simulink model "asm_dfoc"  (R2021a)
settings: Solver=ode23t  StartTime=0.0  StopTime=1  FixedStep=10^(-4)  MaxStep=1e-8  RelTol=1e-3  EnableMultiTasking=on
InitFcn:
  | clear all;
  | P=4;
  | 
  | Rs=28.5e-3;
  | Rr=15.6e-3;
  | 
  | Lm=8e-3;
  | Lls=306e-6;
  | Llr=232e-6;
  | 
  | J=0.805;
  | B=0;%3.5e-2;
  | Ls = Lls+Lm;
  | Lr = Llr+Lm;
  | 
  | Rt = 0.34;
  | u =6.2922;
  | verim=.97
libraries: pid_lib x5, spsdq0toAlphaBetaZeroLib x1
settings Model: Creator=akcan  LastModifiedBy=MSI-
settings SolverCC: AlgebraicLoopSolver=TrustRegion
settings DataIOCC: LimitDataPoints=on  SaveFormat=Array  SignalLoggingSaveFormat=ModelDataLogs  ReturnWorkspaceOutputs=off
settings OptimizationCC: LifeSpan=inf
settings DebuggingCC: UnderspecifiedInitializationDetection=Classic  MergeDetectMultiDrivingBlocksExec=none  SolverPrmCheckMsg=warning  MultiTaskDSMMsg=warning  MultiTaskCondExecSysMsg=none  SFUnexpectedBacktrackingDiag=warning  SFNoUnconditionalDefaultTransitionDiag=warning  SFExecutionAtInitializationDiag=none  SFMachineParentedDataDiag=warning  ArithmeticOperatorsInVariantConditions=warning
settings HardwareCC: ProdBitPerPointer=32  ProdBitPerSizeT=32  ProdBitPerPtrDiffT=32  ProdLargestAtomicFloat=None  ProdIntDivRoundTo=Undefined  ProdEndianess=Unspecified  ProdWordSize=32  ProdHWDeviceType=32-bit Generic
settings ModelReferenceCC: PropagateSignalLabelsOutOfModel=off
settings SFSimCC: SimUseLocalCustomCode=off  CustomCodeUndefinedFunction=UseInterfaceOnly
settings RTWCC: RTWUseLocalCustomCode=off
settings CodeAppCC: StateflowObjectComments=on
settings GRTTargetCC: TargetLangStandard=C89/C90 (ANSI)
settings ConfigComp: CovMetricSettings=dw  CovSaveCumulativeToWorkspaceVar=on  CovSaveSingleToWorkspaceVar=on  CovExternalEMLEnable=off
settings SimscapeCC: SimscapeNormalizeSystem=off

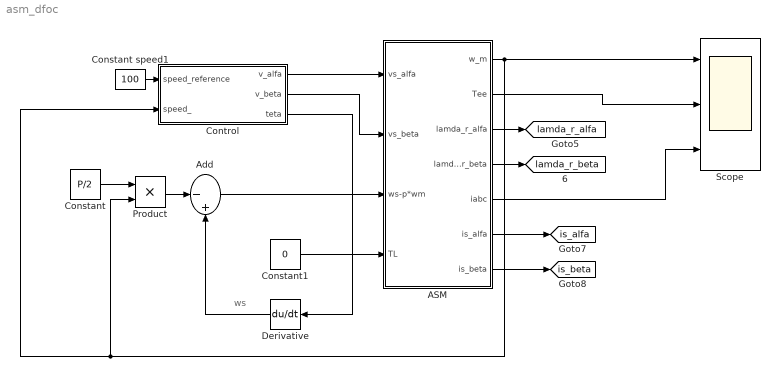
== system asm_dfoc ==
  note: ws
  ASM : Subsystem
  Add : Sum  Inputs=|-+
  Constant : Constant  Value=P/2
  Constant speed1 : Constant  Value=100
  Constant1 : Constant  Value=0
  Control : Subsystem
  Derivative : Derivative
  Product : Product
  Scope : Scope  NumInputPorts=3
  tag scope: is_alfa=global, is_beta=global, lamda_r_alfa=global, lamda_r_beta=global
  wires:
  ASM/3(lamda_r_alfa) -> [lamda_r_alfa]
  ASM/4(lamda_r_beta) -> [lamda_r_beta]
  Control/1("v_alfa ") -> ASM/1(vs_alfa)
  Product/1 -> Add/1
  Constant/1 -> Product/1
  ASM/1(w_m) -> Control/2(speed_), Product/2, Scope/1
  Derivative/1 -> Add/2
  Constant1/1 -> ASM/4(TL)
  Control/2(v_beta) -> ASM/2(vs_beta)
  ASM/7(is_beta) -> [is_beta]
  ASM/6(is_alfa) -> [is_alfa]
  Add/1 -> ASM/3("ws-p*wm ")
  Control/3(teta) -> Derivative/1
  Constant speed1/1 -> Control/1(speed_reference)
  ASM/2(Tee) -> Scope/2
  ASM/5(iabc) -> Scope/3

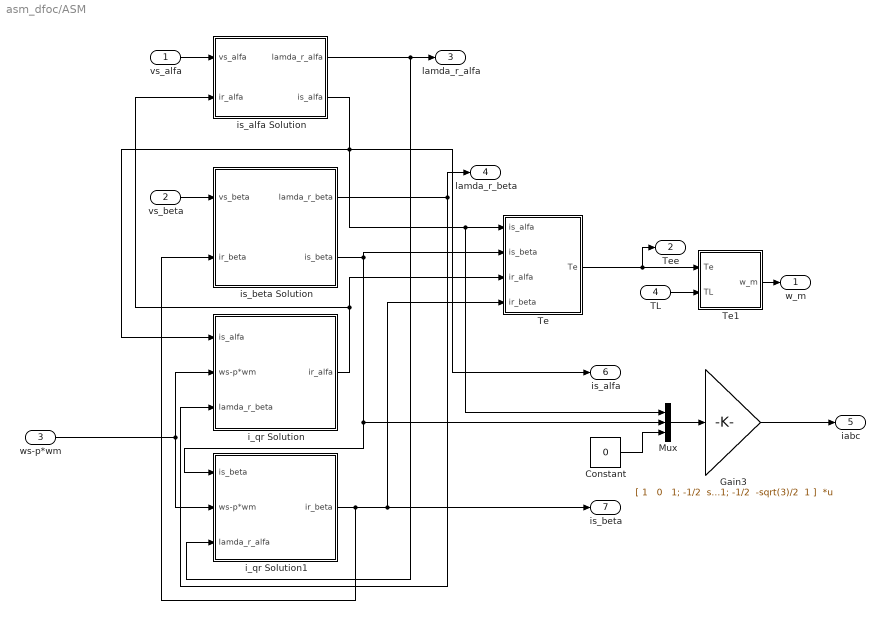
== system asm_dfoc/ASM ==
  vs_alfa : Inport
  vs_beta : Inport  Port=2
  "ws-p*wm " : Inport  Port=3
  TL : Inport  Port=4
  Constant : Constant  Value=0
  Gain3 : Gain  Gain="[ 1   0   1; -1/2  sqrt(3)/2   1; -1/2  -sqrt(3)/2  1 ]"  Multiplication=Matrix(K*u) (u vector)  SaturateOnIntegerOverflow=on  OutDataTypeStr=Inherit: Same as input  ParamDataTypeStr=Inherit: Same as input
  Mux : Mux  Inputs=3
  Te : Subsystem
  Te1 : Subsystem
  i_qr Solution : Subsystem
  i_qr Solution1 : Subsystem
  is_alfa Solution : Subsystem
  is_beta Solution : Subsystem
  w_m : Outport
  Tee : Outport  Port=2
  lamda_r_alfa : Outport  Port=3
  lamda_r_beta : Outport  Port=4
  iabc : Outport  Port=5
  is_alfa : Outport  Port=6
  is_beta : Outport  Port=7
  wires:
  vs_alfa/1 -> is_alfa Solution/1(vs_alfa)
  TL/1 -> Te1/2(TL)
  Te1/1(w_m) -> w_m/1
  Te/1(Te) -> Tee/1, Te1/1(Te)
  vs_beta/1 -> is_beta Solution/1(vs_beta)
  "ws-p*wm "/1 -> i_qr Solution1/2(ws-p*wm), i_qr Solution/2(ws-p*wm)
  Gain3/1 -> iabc/1
  Mux/1 -> Gain3/1
  Constant/1 -> Mux/3
  is_alfa Solution/1(lamda_r_alfa) -> i_qr Solution1/3(lamda_r_alfa), lamda_r_alfa/1
  is_beta Solution/1(lamda_r_beta) -> lamda_r_beta/1, i_qr Solution/3(lamda_r_beta)
  i_qr Solution/1(ir_alfa) -> Te/3(ir_alfa), is_alfa Solution/2(ir_alfa)
  is_beta Solution/2(is_beta) -> Mux/2, i_qr Solution1/1(is_beta), Te/2(is_beta)
  i_qr Solution1/1(ir_beta) -> is_beta/1, Te/4(ir_beta), is_beta Solution/2(ir_beta)
  is_alfa Solution/2(is_alfa) -> is_alfa/1, Mux/1, Te/1(is_alfa), i_qr Solution/1(is_alfa)

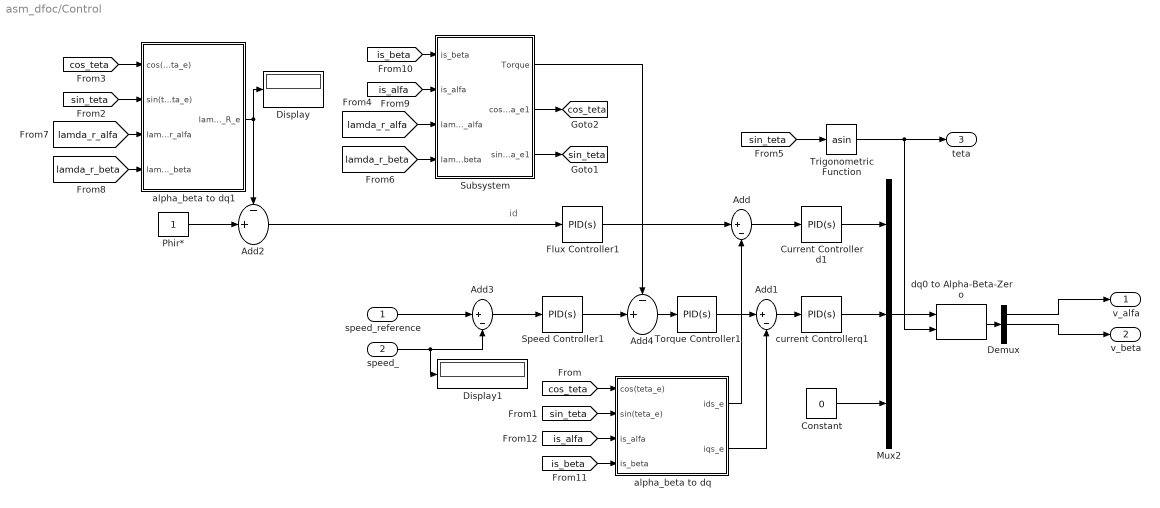
== system asm_dfoc/Control ==
  note: id
  speed_reference : Inport
  speed_ : Inport  Port=2
  Add : Sum  Inputs=|+-
  Add1 : Sum  Inputs=|+-
  Add2 : Sum  Inputs=-+|
  Add3 : Sum  Inputs=|+-
  Add4 : Sum  Inputs=-+|
  Constant : Constant  Value=0
  Current Controller d1 : pid_lib/PID Controller  Controller=PID  Form=Parallel  TimeDomain=Continuous-time  UseExternalTs=off  SampleTime=1  IntegratorMethod=Forward Euler  FilterMethod=Forward Euler  ControllerParametersSource=internal  P=1  I=0.001  D=0  UseFilter=on  N=100  TunerSelectOption=Transfer Function Based (PID Tuner App)  InitialConditionSource=internal  InitialConditionForIntegrator=50  InitialConditionForFilter=0  DifferentiatorICPrevScaledInput=0  ExternalReset=none  TrackingMode=off  Kt=1  LimitOutput=on  SatLimitsSource=internal  UpperSaturationLimit=600  LowerSaturationLimit=-600  LinearizeAsGain=off  AntiWindupMode=clamping  Kb=1  POutMin=[]  POutMax=[]  IOutMin=[]  IOutMax=[]  DOutMin=[]  DOutMax=[]  NOutMin=[]  NOutMax=[]  SumOutMin=[]  SumOutMax=[]  SaturationOutMin=[]  SaturationOutMax=[]  PParamMin=[]  PParamMax=[]  IParamMin=[]  IParamMax=[]  DParamMin=[]  DParamMax=[]  NParamMin=[]  NParamMax=[]  KbParamMin=[]  KbParamMax=[]  KtParamMin=[]  KtParamMax=[]  KbOutMin=[]  KbOutMax=[]  KtOutMin=[]  KtOutMax=[]  IntegratorOutMin=[]  IntegratorOutMax=[]  FilterOutMin=[]  FilterOutMax=[]  SumI1OutMin=[]  SumI1OutMax=[]  SumI2OutMin=[]  SumI2OutMax=[]  SumI3OutMin=[]  SumI3OutMax=[]  SumI4OutMin=[]  SumI4OutMax=[]  SumDOutMin=[]  SumDOutMax=[]  DifferentiatorOutMin=[]  DifferentiatorOutMax=[]  FilterDiffOutCoefMin=[]  FilterDiffOutCoefMax=[]  ReciprocalOutMin=[]  ReciprocalOutMax=[]  SumDenOutMin=[]  SumDenOutMax=[]  SumNumOutMin=[]  SumNumOutMax=[]  DivideOutMin=[]  DivideOutMax=[]  UdiffTsProdOutMin=[]  UdiffTsProdOutMax=[]  NTsProdOutMin=[]  NTsProdOutMax=[]  UintegralTsProdOutMin=[]  UintegralTsProdOutMax=[]  UngainTsProdOutMin=[]  UngainTsProdOutMax=[]  IntegratorContinuousStateAttributes=''  IntegratorStateMustResolveToSignalObject=off  IntegratorRTWStateStorageClass=Auto  FilterContinuousStateAttributes=''  FilterStateMustResolveToSignalObject=off  FilterRTWStateStorageClass=Auto  ParallelPVariant=InternalParameters  IdealPVariant=Disabled  IVariant=InternalParameters  DVariant=InternalParameters  IntegratorVariant=Continuous  SatVariant=Enabled  AWVariant=ContClampingParallel  PCopyVariant=Disabled  TRVariant=Disabled  FdbkBlocksVariant=Forward  IdealPFdbkVariant=Disabled  SatFdbkVariant=Disabled  DerivativeFilterVariant=ContFilter  NVariant=InternalParameters  NCopyVariant=Disabled  FilterICVariant=InternalICsFilter  IntegratorICVariant=InternalICs  ExternalResetVariant=Disabled  TRSumVariant=Passthrough  SumFdbkVariant=Disabled  SumVariant=Sum_PID  TsampFilterVariant=InternalTs  TsampNgainVariant=Passthrough  TsampIntegralVariant=Passthrough  ExternalSaturationOutDataTypeStr=Inherit: Same as second input
  Demux : Demux  Outputs=3
  Display : Display
  Display1 : Display
  Flux Controller1 : pid_lib/PID Controller  Controller=PID  Form=Parallel  TimeDomain=Continuous-time  UseExternalTs=off  SampleTime=1  IntegratorMethod=Forward Euler  FilterMethod=Forward Euler  ControllerParametersSource=internal  P=1  I=0.001  D=0  UseFilter=on  N=100  TunerSelectOption=Transfer Function Based (PID Tuner App)  InitialConditionSource=internal  InitialConditionForIntegrator=100  InitialConditionForFilter=0  DifferentiatorICPrevScaledInput=0  ExternalReset=none  TrackingMode=off  Kt=1  LimitOutput=on  SatLimitsSource=internal  UpperSaturationLimit=300  LowerSaturationLimit=-300  LinearizeAsGain=off  AntiWindupMode=clamping  Kb=1  POutMin=[]  POutMax=[]  IOutMin=[]  IOutMax=[]  DOutMin=[]  DOutMax=[]  NOutMin=[]  NOutMax=[]  SumOutMin=[]  SumOutMax=[]  SaturationOutMin=[]  SaturationOutMax=[]  PParamMin=[]  PParamMax=[]  IParamMin=[]  IParamMax=[]  DParamMin=[]  DParamMax=[]  NParamMin=[]  NParamMax=[]  KbParamMin=[]  KbParamMax=[]  KtParamMin=[]  KtParamMax=[]  KbOutMin=[]  KbOutMax=[]  KtOutMin=[]  KtOutMax=[]  IntegratorOutMin=[]  IntegratorOutMax=[]  FilterOutMin=[]  FilterOutMax=[]  SumI1OutMin=[]  SumI1OutMax=[]  SumI2OutMin=[]  SumI2OutMax=[]  SumI3OutMin=[]  SumI3OutMax=[]  SumI4OutMin=[]  SumI4OutMax=[]  SumDOutMin=[]  SumDOutMax=[]  DifferentiatorOutMin=[]  DifferentiatorOutMax=[]  FilterDiffOutCoefMin=[]  FilterDiffOutCoefMax=[]  ReciprocalOutMin=[]  ReciprocalOutMax=[]  SumDenOutMin=[]  SumDenOutMax=[]  SumNumOutMin=[]  SumNumOutMax=[]  DivideOutMin=[]  DivideOutMax=[]  UdiffTsProdOutMin=[]  UdiffTsProdOutMax=[]  NTsProdOutMin=[]  NTsProdOutMax=[]  UintegralTsProdOutMin=[]  UintegralTsProdOutMax=[]  UngainTsProdOutMin=[]  UngainTsProdOutMax=[]  IntegratorContinuousStateAttributes=''  IntegratorStateMustResolveToSignalObject=off  IntegratorRTWStateStorageClass=Auto  FilterContinuousStateAttributes=''  FilterStateMustResolveToSignalObject=off  FilterRTWStateStorageClass=Auto  ParallelPVariant=InternalParameters  IdealPVariant=Disabled  IVariant=InternalParameters  DVariant=InternalParameters  IntegratorVariant=Continuous  SatVariant=Enabled  AWVariant=ContClampingParallel  PCopyVariant=Disabled  TRVariant=Disabled  FdbkBlocksVariant=Forward  IdealPFdbkVariant=Disabled  SatFdbkVariant=Disabled  DerivativeFilterVariant=ContFilter  NVariant=InternalParameters  NCopyVariant=Disabled  FilterICVariant=InternalICsFilter  IntegratorICVariant=InternalICs  ExternalResetVariant=Disabled  TRSumVariant=Passthrough  SumFdbkVariant=Disabled  SumVariant=Sum_PID  TsampFilterVariant=InternalTs  TsampNgainVariant=Passthrough  TsampIntegralVariant=Passthrough  ExternalSaturationOutDataTypeStr=Inherit: Same as second input
  Mux2 : Mux  Inputs=3
  Phir* : Constant
  Speed Controller1 : pid_lib/PID Controller  Controller=PID  Form=Parallel  TimeDomain=Continuous-time  UseExternalTs=off  SampleTime=1  IntegratorMethod=Forward Euler  FilterMethod=Forward Euler  ControllerParametersSource=internal  P=1  I=0.01  D=0  UseFilter=on  N=100  TunerSelectOption=Transfer Function Based (PID Tuner App)  InitialConditionSource=internal  InitialConditionForIntegrator=100  InitialConditionForFilter=0  DifferentiatorICPrevScaledInput=0  ExternalReset=none  TrackingMode=off  Kt=1  LimitOutput=off  SatLimitsSource=internal  UpperSaturationLimit=200  LowerSaturationLimit=-200  LinearizeAsGain=off  AntiWindupMode=clamping  Kb=1  POutMin=[]  POutMax=[]  IOutMin=[]  IOutMax=[]  DOutMin=[]  DOutMax=[]  NOutMin=[]  NOutMax=[]  SumOutMin=[]  SumOutMax=[]  SaturationOutMin=[]  SaturationOutMax=[]  PParamMin=[]  PParamMax=[]  IParamMin=[]  IParamMax=[]  DParamMin=[]  DParamMax=[]  NParamMin=[]  NParamMax=[]  KbParamMin=[]  KbParamMax=[]  KtParamMin=[]  KtParamMax=[]  KbOutMin=[]  KbOutMax=[]  KtOutMin=[]  KtOutMax=[]  IntegratorOutMin=[]  IntegratorOutMax=[]  FilterOutMin=[]  FilterOutMax=[]  SumI1OutMin=[]  SumI1OutMax=[]  SumI2OutMin=[]  SumI2OutMax=[]  SumI3OutMin=[]  SumI3OutMax=[]  SumI4OutMin=[]  SumI4OutMax=[]  SumDOutMin=[]  SumDOutMax=[]  DifferentiatorOutMin=[]  DifferentiatorOutMax=[]  FilterDiffOutCoefMin=[]  FilterDiffOutCoefMax=[]  ReciprocalOutMin=[]  ReciprocalOutMax=[]  SumDenOutMin=[]  SumDenOutMax=[]  SumNumOutMin=[]  SumNumOutMax=[]  DivideOutMin=[]  DivideOutMax=[]  UdiffTsProdOutMin=[]  UdiffTsProdOutMax=[]  NTsProdOutMin=[]  NTsProdOutMax=[]  UintegralTsProdOutMin=[]  UintegralTsProdOutMax=[]  UngainTsProdOutMin=[]  UngainTsProdOutMax=[]  IntegratorContinuousStateAttributes=''  IntegratorStateMustResolveToSignalObject=off  IntegratorRTWStateStorageClass=Auto  FilterContinuousStateAttributes=''  FilterStateMustResolveToSignalObject=off  FilterRTWStateStorageClass=Auto  ParallelPVariant=InternalParameters  IdealPVariant=Disabled  IVariant=InternalParameters  DVariant=InternalParameters  IntegratorVariant=Continuous  SatVariant=Disabled  AWVariant=Passthrough  PCopyVariant=Disabled  TRVariant=Disabled  FdbkBlocksVariant=Forward  IdealPFdbkVariant=Disabled  SatFdbkVariant=Disabled  DerivativeFilterVariant=ContFilter  NVariant=InternalParameters  NCopyVariant=Disabled  FilterICVariant=InternalICsFilter  IntegratorICVariant=InternalICs  ExternalResetVariant=Disabled  TRSumVariant=Passthrough  SumFdbkVariant=Disabled  SumVariant=Sum_PID  TsampFilterVariant=InternalTs  TsampNgainVariant=Passthrough  TsampIntegralVariant=Passthrough  ExternalSaturationOutDataTypeStr=Inherit: Same as second input
  Subsystem : Subsystem
  Torque Controller1 : pid_lib/PID Controller  Controller=PID  Form=Parallel  TimeDomain=Continuous-time  UseExternalTs=off  SampleTime=1  IntegratorMethod=Forward Euler  FilterMethod=Forward Euler  ControllerParametersSource=internal  P=1  I=0.01  D=0  UseFilter=on  N=100  TunerSelectOption=Transfer Function Based (PID Tuner App)  InitialConditionSource=internal  InitialConditionForIntegrator=50  InitialConditionForFilter=0  DifferentiatorICPrevScaledInput=0  ExternalReset=none  TrackingMode=off  Kt=1  LimitOutput=on  SatLimitsSource=internal  UpperSaturationLimit=300  LowerSaturationLimit=-300  LinearizeAsGain=off  AntiWindupMode=clamping  Kb=1  POutMin=[]  POutMax=[]  IOutMin=[]  IOutMax=[]  DOutMin=[]  DOutMax=[]  NOutMin=[]  NOutMax=[]  SumOutMin=[]  SumOutMax=[]  SaturationOutMin=[]  SaturationOutMax=[]  PParamMin=[]  PParamMax=[]  IParamMin=[]  IParamMax=[]  DParamMin=[]  DParamMax=[]  NParamMin=[]  NParamMax=[]  KbParamMin=[]  KbParamMax=[]  KtParamMin=[]  KtParamMax=[]  KbOutMin=[]  KbOutMax=[]  KtOutMin=[]  KtOutMax=[]  IntegratorOutMin=[]  IntegratorOutMax=[]  FilterOutMin=[]  FilterOutMax=[]  SumI1OutMin=[]  SumI1OutMax=[]  SumI2OutMin=[]  SumI2OutMax=[]  SumI3OutMin=[]  SumI3OutMax=[]  SumI4OutMin=[]  SumI4OutMax=[]  SumDOutMin=[]  SumDOutMax=[]  DifferentiatorOutMin=[]  DifferentiatorOutMax=[]  FilterDiffOutCoefMin=[]  FilterDiffOutCoefMax=[]  ReciprocalOutMin=[]  ReciprocalOutMax=[]  SumDenOutMin=[]  SumDenOutMax=[]  SumNumOutMin=[]  SumNumOutMax=[]  DivideOutMin=[]  DivideOutMax=[]  UdiffTsProdOutMin=[]  UdiffTsProdOutMax=[]  NTsProdOutMin=[]  NTsProdOutMax=[]  UintegralTsProdOutMin=[]  UintegralTsProdOutMax=[]  UngainTsProdOutMin=[]  UngainTsProdOutMax=[]  IntegratorContinuousStateAttributes=''  IntegratorStateMustResolveToSignalObject=off  IntegratorRTWStateStorageClass=Auto  FilterContinuousStateAttributes=''  FilterStateMustResolveToSignalObject=off  FilterRTWStateStorageClass=Auto  ParallelPVariant=InternalParameters  IdealPVariant=Disabled  IVariant=InternalParameters  DVariant=InternalParameters  IntegratorVariant=Continuous  SatVariant=Enabled  AWVariant=ContClampingParallel  PCopyVariant=Disabled  TRVariant=Disabled  FdbkBlocksVariant=Forward  IdealPFdbkVariant=Disabled  SatFdbkVariant=Disabled  DerivativeFilterVariant=ContFilter  NVariant=InternalParameters  NCopyVariant=Disabled  FilterICVariant=InternalICsFilter  IntegratorICVariant=InternalICs  ExternalResetVariant=Disabled  TRSumVariant=Passthrough  SumFdbkVariant=Disabled  SumVariant=Sum_PID  TsampFilterVariant=InternalTs  TsampNgainVariant=Passthrough  TsampIntegralVariant=Passthrough  ExternalSaturationOutDataTypeStr=Inherit: Same as second input
  Trigonometric Function : Trigonometry  Operator=asin
  alpha_beta to dq : Subsystem
  alpha_beta to dq1 : Subsystem
  current Controllerq1 : pid_lib/PID Controller  Controller=PID  Form=Parallel  TimeDomain=Continuous-time  UseExternalTs=off  SampleTime=1  IntegratorMethod=Forward Euler  FilterMethod=Forward Euler  ControllerParametersSource=internal  P=1  I=0.01  D=0  UseFilter=on  N=100  TunerSelectOption=Transfer Function Based (PID Tuner App)  InitialConditionSource=internal  InitialConditionForIntegrator=50  InitialConditionForFilter=0  DifferentiatorICPrevScaledInput=0  ExternalReset=none  TrackingMode=off  Kt=1  LimitOutput=on  SatLimitsSource=internal  UpperSaturationLimit=600  LowerSaturationLimit=-600  LinearizeAsGain=off  AntiWindupMode=clamping  Kb=1  POutMin=[]  POutMax=[]  IOutMin=[]  IOutMax=[]  DOutMin=[]  DOutMax=[]  NOutMin=[]  NOutMax=[]  SumOutMin=[]  SumOutMax=[]  SaturationOutMin=[]  SaturationOutMax=[]  PParamMin=[]  PParamMax=[]  IParamMin=[]  IParamMax=[]  DParamMin=[]  DParamMax=[]  NParamMin=[]  NParamMax=[]  KbParamMin=[]  KbParamMax=[]  KtParamMin=[]  KtParamMax=[]  KbOutMin=[]  KbOutMax=[]  KtOutMin=[]  KtOutMax=[]  IntegratorOutMin=[]  IntegratorOutMax=[]  FilterOutMin=[]  FilterOutMax=[]  SumI1OutMin=[]  SumI1OutMax=[]  SumI2OutMin=[]  SumI2OutMax=[]  SumI3OutMin=[]  SumI3OutMax=[]  SumI4OutMin=[]  SumI4OutMax=[]  SumDOutMin=[]  SumDOutMax=[]  DifferentiatorOutMin=[]  DifferentiatorOutMax=[]  FilterDiffOutCoefMin=[]  FilterDiffOutCoefMax=[]  ReciprocalOutMin=[]  ReciprocalOutMax=[]  SumDenOutMin=[]  SumDenOutMax=[]  SumNumOutMin=[]  SumNumOutMax=[]  DivideOutMin=[]  DivideOutMax=[]  UdiffTsProdOutMin=[]  UdiffTsProdOutMax=[]  NTsProdOutMin=[]  NTsProdOutMax=[]  UintegralTsProdOutMin=[]  UintegralTsProdOutMax=[]  UngainTsProdOutMin=[]  UngainTsProdOutMax=[]  IntegratorContinuousStateAttributes=''  IntegratorStateMustResolveToSignalObject=off  IntegratorRTWStateStorageClass=Auto  FilterContinuousStateAttributes=''  FilterStateMustResolveToSignalObject=off  FilterRTWStateStorageClass=Auto  ParallelPVariant=InternalParameters  IdealPVariant=Disabled  IVariant=InternalParameters  DVariant=InternalParameters  IntegratorVariant=Continuous  SatVariant=Enabled  AWVariant=ContClampingParallel  PCopyVariant=Disabled  TRVariant=Disabled  FdbkBlocksVariant=Forward  IdealPFdbkVariant=Disabled  SatFdbkVariant=Disabled  DerivativeFilterVariant=ContFilter  NVariant=InternalParameters  NCopyVariant=Disabled  FilterICVariant=InternalICsFilter  IntegratorICVariant=InternalICs  ExternalResetVariant=Disabled  TRSumVariant=Passthrough  SumFdbkVariant=Disabled  SumVariant=Sum_PID  TsampFilterVariant=InternalTs  TsampNgainVariant=Passthrough  TsampIntegralVariant=Passthrough  ExternalSaturationOutDataTypeStr=Inherit: Same as second input
  dq0 to Alpha-Beta-Zero : spsdq0toAlphaBetaZeroLib/dq0 to Alpha-Beta-Zero  Alignment=Aligned with phase A axis
      settings: SourceProductBaseCode=PS
  "v_alfa " : Outport
  v_beta : Outport  Port=2
  teta : Outport  Port=3
  tag scope: cos_teta=global, sin_teta=global
  wires:
  Demux/2 -> v_beta/1
  Phir*/1 -> Add2/2
  Add4/1 -> Torque Controller1/1
  Add2/1 -> Flux Controller1/1
  speed_reference/1 -> Add3/1
  Speed Controller1/1 -> Add4/2
  Add/1 -> Current Controller d1/1
  Add1/1 -> current Controllerq1/1
  Mux2/1 -> dq0 to Alpha-Beta-Zero/1
  Constant/1 -> Mux2/3
  dq0 to Alpha-Beta-Zero/1 -> Demux/1
  Demux/1 -> "v_alfa "/1
  Trigonometric Function/1 -> teta/1, dq0 to Alpha-Beta-Zero/2
  alpha_beta to dq1/1("lamda_R_e ") -> Add2/1, Display/1
  alpha_beta to dq/1("ids_e ") -> Add/2
  alpha_beta to dq/2(iqs_e) -> Add1/2
  Flux Controller1/1 -> Add/1
  Torque Controller1/1 -> Add1/1
  Current Controller d1/1 -> Mux2/1
  current Controllerq1/1 -> Mux2/2
  Subsystem/3(sin_teta_e1) -> [sin_teta]
  Subsystem/2(cos_teta_e1) -> [cos_teta]
  [cos_teta] -> alpha_beta to dq/1(cos(teta_e))
  [sin_teta] -> alpha_beta to dq/2(sin(teta_e))
  [sin_teta] -> alpha_beta to dq1/2(sin(teta_e))
  [cos_teta] -> alpha_beta to dq1/1(cos(teta_e))
  [lamda_r_alfa] -> Subsystem/3("lamda_r_alfa ")
  [sin_teta] -> Trigonometric Function/1
  [lamda_r_beta] -> Subsystem/4(lamda_r_beta)
  [lamda_r_alfa] -> alpha_beta to dq1/3(lamda_r_alfa)
  [lamda_r_beta] -> alpha_beta to dq1/4(lamda_r_beta)
  [is_alfa] -> Subsystem/2(is_alfa)
  [is_beta] -> Subsystem/1(is_beta)
  [is_beta] -> alpha_beta to dq/4(is_beta)
  [is_alfa] -> alpha_beta to dq/3(is_alfa)
  speed_/1 -> Display1/1, Add3/2
  Add3/1 -> Speed Controller1/1
  Subsystem/1(Torque) -> Add4/1

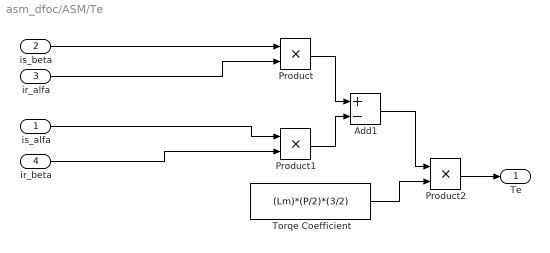
== system asm_dfoc/ASM/Te ==
  is_alfa : Inport
  is_beta : Inport  Port=2
  ir_alfa : Inport  Port=3
  ir_beta : Inport  Port=4
  Add1 : Sum  Inputs=+-
  Product : Product
  Product1 : Product
  Product2 : Product
  Torqe Coefficient : Constant  Value=(Lm)*(P/2)*(3/2)
  Te : Outport
  wires:
  Product/1 -> Add1/1
  Product1/1 -> Add1/2
  Add1/1 -> Product2/1
  Torqe Coefficient/1 -> Product2/2
  Product2/1 -> Te/1
  is_beta/1 -> Product/1
  ir_alfa/1 -> Product/2
  is_alfa/1 -> Product1/1
  ir_beta/1 -> Product1/2

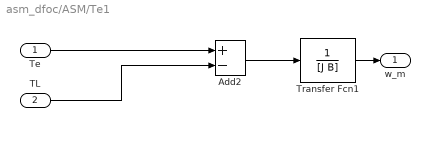
== system asm_dfoc/ASM/Te1 ==
  Te : Inport
  TL : Inport  Port=2
  Add2 : Sum  Inputs=+-
  Transfer Fcn1 : TransferFcn  Denominator=[J B]
  w_m : Outport
  wires:
  Add2/1 -> Transfer Fcn1/1
  Transfer Fcn1/1 -> w_m/1
  Te/1 -> Add2/1
  TL/1 -> Add2/2

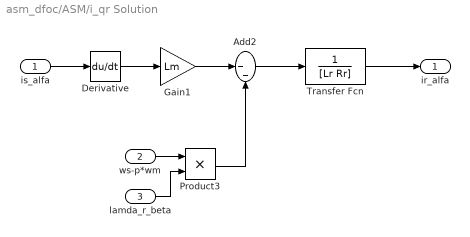
== system asm_dfoc/ASM/i_qr Solution ==
  is_alfa : Inport
  ws-p*wm : Inport  Port=2
  lamda_r_beta : Inport  Port=3
  Add2 : Sum  Inputs=|--
  Derivative : Derivative
  Gain1 : Gain  Gain=Lm
  Product3 : Product
  Transfer Fcn : TransferFcn  Denominator=[Lr Rr]
  ir_alfa : Outport
  wires:
  is_alfa/1 -> Derivative/1
  Derivative/1 -> Gain1/1
  Gain1/1 -> Add2/1
  Product3/1 -> Add2/2
  ws-p*wm/1 -> Product3/1
  lamda_r_beta/1 -> Product3/2
  Add2/1 -> Transfer Fcn/1
  Transfer Fcn/1 -> ir_alfa/1

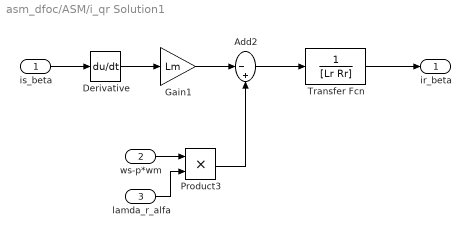
== system asm_dfoc/ASM/i_qr Solution1 ==
  is_beta : Inport
  ws-p*wm : Inport  Port=2
  lamda_r_alfa : Inport  Port=3
  Add2 : Sum  Inputs=|-+
  Derivative : Derivative
  Gain1 : Gain  Gain=Lm
  Product3 : Product
  Transfer Fcn : TransferFcn  Denominator=[Lr Rr]
  ir_beta : Outport
  wires:
  is_beta/1 -> Derivative/1
  Derivative/1 -> Gain1/1
  Gain1/1 -> Add2/1
  Product3/1 -> Add2/2
  ws-p*wm/1 -> Product3/1
  lamda_r_alfa/1 -> Product3/2
  Add2/1 -> Transfer Fcn/1
  Transfer Fcn/1 -> ir_beta/1

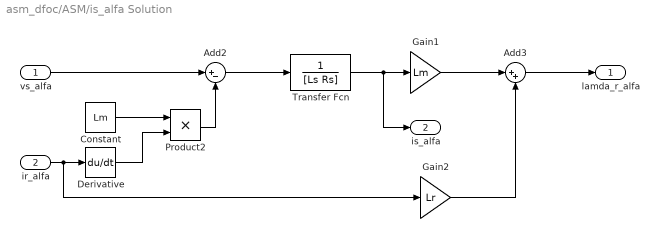
== system asm_dfoc/ASM/is_alfa Solution ==
  vs_alfa : Inport
  ir_alfa : Inport  Port=2
  Add2 : Sum  Inputs=|+-
  Add3 : Sum  Inputs=|++
  Constant : Constant  Value=Lm
  Derivative : Derivative
  Gain1 : Gain  Gain=Lm
  Gain2 : Gain  Gain=Lr
  Product2 : Product
  Transfer Fcn : TransferFcn  Denominator=[Ls Rs]
  lamda_r_alfa : Outport
  is_alfa : Outport  Port=2
  wires:
  vs_alfa/1 -> Add2/1
  Product2/1 -> Add2/2
  Add2/1 -> Transfer Fcn/1
  Transfer Fcn/1 -> Gain1/1, is_alfa/1
  Constant/1 -> Product2/1
  ir_alfa/1 -> Gain2/1, Derivative/1
  Derivative/1 -> Product2/2
  Gain1/1 -> Add3/1
  Gain2/1 -> Add3/2
  Add3/1 -> lamda_r_alfa/1

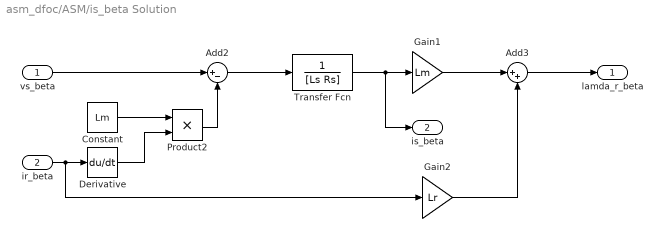
== system asm_dfoc/ASM/is_beta Solution ==
  vs_beta : Inport
  ir_beta : Inport  Port=2
  Add2 : Sum  Inputs=|+-
  Add3 : Sum  Inputs=|++
  Constant : Constant  Value=Lm
  Derivative : Derivative
  Gain1 : Gain  Gain=Lm
  Gain2 : Gain  Gain=Lr
  Product2 : Product
  Transfer Fcn : TransferFcn  Denominator=[Ls Rs]
  lamda_r_beta : Outport
  is_beta : Outport  Port=2
  wires:
  vs_beta/1 -> Add2/1
  Product2/1 -> Add2/2
  Add2/1 -> Transfer Fcn/1
  Transfer Fcn/1 -> Gain1/1, is_beta/1
  Constant/1 -> Product2/1
  ir_beta/1 -> Gain2/1, Derivative/1
  Derivative/1 -> Product2/2
  Gain1/1 -> Add3/1
  Gain2/1 -> Add3/2
  Add3/1 -> lamda_r_beta/1

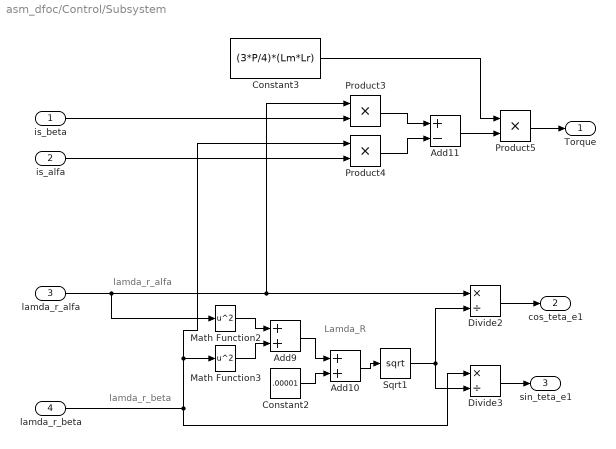
== system asm_dfoc/Control/Subsystem ==
  note: lamda_r_beta
  note: lamda_r_alfa
  note: Lamda_R
  is_beta : Inport
  is_alfa : Inport  Port=2
  "lamda_r_alfa " : Inport  Port=3
  lamda_r_beta : Inport  Port=4
  Add10 : Sum
  Add11 : Sum  Inputs=+-
  Add9 : Sum
  Constant2 : Constant  Value=.00001
  Constant3 : Constant  Value=(3*P/4)*(Lm*Lr)
  Divide2 : Product  Inputs=*/
  Divide3 : Product  Inputs=*/
  Math Function2 : Math  Operator=square  SignedPower=on  SaturateOnIntegerOverflow=on
  Math Function3 : Math  Operator=square  SignedPower=on  SaturateOnIntegerOverflow=on
  Product3 : Product
  Product4 : Product
  Product5 : Product
  Sqrt1 : Sqrt  SaturateOnIntegerOverflow=on
  Torque : Outport
  cos_teta_e1 : Outport  Port=2
  sin_teta_e1 : Outport  Port=3
  wires:
  is_beta/1 -> Product3/2
  is_alfa/1 -> Product4/2
  Math Function2/1 -> Add9/1
  Math Function3/1 -> Add9/2
  Add9/1 -> Add10/1
  Add10/1 -> Sqrt1/1
  Constant2/1 -> Add10/2
  "lamda_r_alfa "/1 -> Divide2/1, Product3/1, Math Function2/1
  lamda_r_beta/1 -> Product4/1, Math Function3/1, Divide3/1
  Divide2/1 -> cos_teta_e1/1
  Divide3/1 -> sin_teta_e1/1
  Sqrt1/1 -> Divide3/2, Divide2/2
  Product3/1 -> Add11/1
  Add11/1 -> Product5/2
  Constant3/1 -> Product5/1
  Product4/1 -> Add11/2
  Product5/1 -> Torque/1

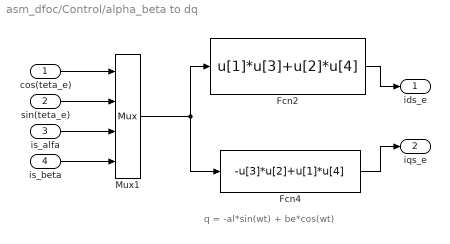
== system asm_dfoc/Control/alpha_beta to dq ==
  note: q = -al*sin(wt) + be*cos(wt)
  cos(teta_e) : Inport
  sin(teta_e) : Inport  Port=2
  is_alfa : Inport  Port=3
  is_beta : Inport  Port=4
  Fcn2 : Fcn  Expr=u[1]*u[3]+u[2]*u[4]
  Fcn4 : Fcn  Expr=-u[3]*u[2]+u[1]*u[4]
  Mux1 : Mux
  "ids_e " : Outport
  iqs_e : Outport  Port=2
  wires:
  Mux1/1 -> Fcn4/1, Fcn2/1
  is_beta/1 -> Mux1/4
  cos(teta_e)/1 -> Mux1/1
  Fcn2/1 -> "ids_e "/1
  Fcn4/1 -> iqs_e/1
  sin(teta_e)/1 -> Mux1/2
  is_alfa/1 -> Mux1/3

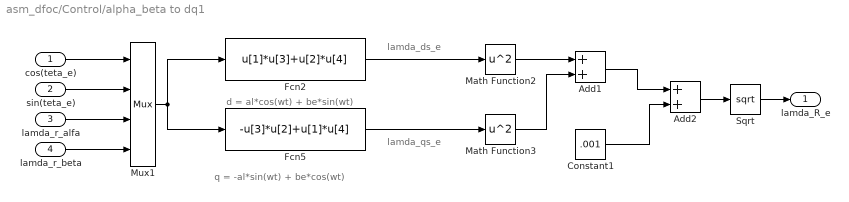
== system asm_dfoc/Control/alpha_beta to dq1 ==
  note: lamda_ds_e
  note: lamda_qs_e
  note: d = al*cos(wt) + be*sin(wt)
  note: q = -al*sin(wt) + be*cos(wt)
  cos(teta_e) : Inport
  sin(teta_e) : Inport  Port=2
  lamda_r_alfa : Inport  Port=3
  lamda_r_beta : Inport  Port=4
  Add1 : Sum
  Add2 : Sum
  Constant1 : Constant  Value=.001
  Fcn2 : Fcn  Expr=u[1]*u[3]+u[2]*u[4]
  Fcn5 : Fcn  Expr=-u[3]*u[2]+u[1]*u[4]
  Math Function2 : Math  Operator=square  SignedPower=on  SaturateOnIntegerOverflow=on
  Math Function3 : Math  Operator=square  SignedPower=on  SaturateOnIntegerOverflow=on
  Mux1 : Mux
  Sqrt : Sqrt  SaturateOnIntegerOverflow=on
  "lamda_R_e " : Outport
  wires:
  cos(teta_e)/1 -> Mux1/1
  Sqrt/1 -> "lamda_R_e "/1
  Constant1/1 -> Add2/2
  Fcn2/1 -> Math Function2/1
  Math Function2/1 -> Add1/1
  Fcn5/1 -> Math Function3/1
  Add1/1 -> Add2/1
  Math Function3/1 -> Add1/2
  Add2/1 -> Sqrt/1
  lamda_r_alfa/1 -> Mux1/3
  lamda_r_beta/1 -> Mux1/4
  Mux1/1 -> Fcn2/1, Fcn5/1
  sin(teta_e)/1 -> Mux1/2
